simulink library "NSA_DEVS_LOGISTICS_COUPLED"  (R2023a)
settings: Solver=VariableStepAuto  StartTime=0.0  StopTime=10.0  RelTol=1e-3
libraries: NSA_DEVS_LOGISTICS_ATOMIC x3, NSA_DEVS_DIGITAL_LOGIC_ATOMIC x2, NSA_DEVS_MATH_OPERATIONS_ATOMIC x1
settings Model: Creator=david  LastModifiedBy=peter

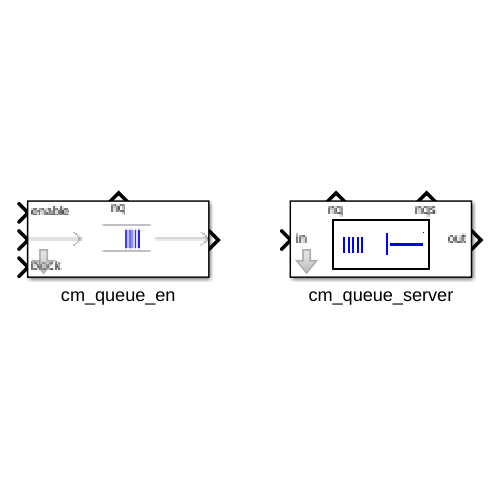
[thumbnail: Simulink's stored preview of the top-level diagram]
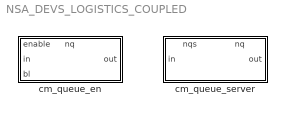
== system NSA_DEVS_LOGISTICS_COUPLED ==
  cm_queue_en : Subsystem  mask{tau=[0,1], debug=0}
      settings: PortSchema="{\"entries\":[{\"content\":{\"sides\":[{\"content\":{\"connectorIds\":[\"In1\",\"In2\",\"In3\"]},\"type\":\"ConnectorPlacement.EquallySpacedRectSide\",\"uuid\":\"049aff47-2d52-45a1-8cfe-c5a626c266e1\"},{\"content\":{\"connectorIds\":[\"Out1\"],\"side\":\"RIGHT\"},\"type\":\"ConnectorPlacement.EquallySpacedRectSide\",\"uuid\":\"d161dc95-73c9-457a-a499-61ffb49d079d\"},{\"content\":{\"connectorIds\":[\"Out2\"],\"side\":\"TOP\"},\"type\":\"ConnectorPlacement.EquallySpacedRectSide\",\"uuid\":\"1785de47-7f68-4a9a-b5e6-0a66b4c3b55d\"}]},\"type\":\"ConnectorPlacement.EquallySpacedConnector\",\"uuid\":\"6ecdd4d2-0921-4324-b437-891f6fdb2f7e\"}],\"packageUris\":[\"http://schema.mathworks.com/mf0/Connector/R2020b\"],\"version\":\"1.0\"}"
  cm_queue_server : Subsystem  mask{ts=1.0, tau=[0,1], debug=0}
      settings: PortSchema="{\"entries\":[{\"content\":{\"sides\":[{\"content\":{\"connectorIds\":[\"In1\"]},\"type\":\"ConnectorPlacement.EquallySpacedRectSide\",\"uuid\":\"07fa0e51-8843-4ac9-8e94-884ae9a89d36\"},{\"content\":{\"connectorIds\":[\"Out1\"],\"side\":\"RIGHT\"},\"type\":\"ConnectorPlacement.EquallySpacedRectSide\",\"uuid\":\"0131ce69-7449-4362-9cfd-88c0df269334\"},{\"content\":{\"connectorIds\":[\"Out2\",\"Out3\"],\"side\":\"TOP\"},\"type\":\"ConnectorPlacement.EquallySpacedRectSide\",\"uuid\":\"407e2fdf-9916-4f3f-84c2-2a472bd1d59f\"}]},\"type\":\"ConnectorPlacement.EquallySpacedConnector\",\"uuid\":\"291a1c46-4425-425c-bba8-593c7bd17cc2\"}],\"packageUris\":[\"http://schema.mathworks.com/mf0/Connector/R2020b\"],\"version\":\"1.0\"}"
      mask DialogControl Container4 Prompt: General
      mask DialogControl Container5 Prompt: Advanced

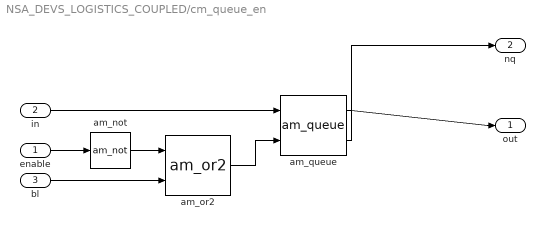
== system NSA_DEVS_LOGISTICS_COUPLED/cm_queue_en ==
  enable : Inport
  in : Inport  Port=2
  bl : Inport  Port=3
  am_not : NSA_DEVS_DIGITAL_LOGIC_ATOMIC/am_not  tau=[0,1]  debug=0
      settings: SourceProductName=NSA_DEVS
  am_or2 : NSA_DEVS_DIGITAL_LOGIC_ATOMIC/am_or2  tau=[0,1]  debug=0
      settings: SourceProductName=NSA_DEVS
  am_queue : NSA_DEVS_LOGISTICS_ATOMIC/am_queue  tD=tau+[0,1]  tau=tau  debug=debug
      settings: SourceProductName=NSA_DEVS
  out : Outport
  nq : Outport  Port=2
  wires:
  in/1 -> am_queue/1
  am_queue/1 -> out/1
  am_queue/2 -> nq/1
  enable/1 -> am_not/1
  bl/1 -> am_or2/2
  am_not/1 -> am_or2/1
  am_or2/1 -> am_queue/2

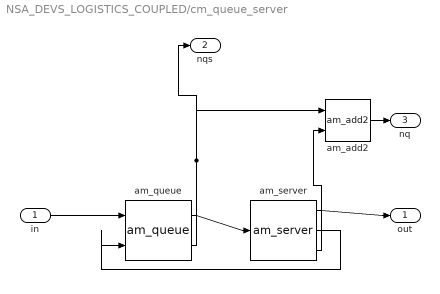
== system NSA_DEVS_LOGISTICS_COUPLED/cm_queue_server ==
  in : Inport
  am_add2 : NSA_DEVS_MATH_OPERATIONS_ATOMIC/am_add2  tau=tau  debug=debug
      settings: SourceProductName=NSA_DEVS
  am_queue : NSA_DEVS_LOGISTICS_ATOMIC/am_queue  tD=tau.*2  tau=tau  debug=debug
      settings: SourceProductName=NSA_DEVS
  am_server : NSA_DEVS_LOGISTICS_ATOMIC/am_server  tS=ts  tau=tau  debug=debug
      settings: SourceProductName=NSA_DEVS
  out : Outport
  nqs : Outport  Port=2
  nq : Outport  Port=3
  wires:
  am_queue/1 -> am_server/1
  in/1 -> am_queue/1
  am_server/2 -> am_queue/2
  am_server/1 -> out/1
  am_queue/2 -> am_add2/1, nqs/1
  am_server/3 -> am_add2/2
  am_add2/1 -> nq/1
